simulink model "TP2"  (R2024b)
settings: Solver=VariableStepAuto  StartTime=0.0  StopTime=10  RelTol=1e-3
InitFcn:
  | J=0.28 %kg.m2.s-2
  | b=8.5e-3 %N.m.s
  | K=0.5093 %N.m.A-1
  | R=0.13 %Omh
  | L=1.6e-3 %H
  | Cr=0 %N.m
  | U=12 %V
  | v=2 %m.s-1
  | Kpos=1
StartFcn:
  | J=0.28 %kg.m2.s-2
  | b=8.5e-3 %N.m.s
  | K=0.5093 %N.m.A-1
  | R=0.13 %Omh
  | L=1.6e-3 %H
  | Cr=0 %N.m
  | U=12 %V
  | v=2 %m.s-1
  | Kpos=1
settings Model: Creator=E306-PC5  LastModifiedBy=E306-PC5

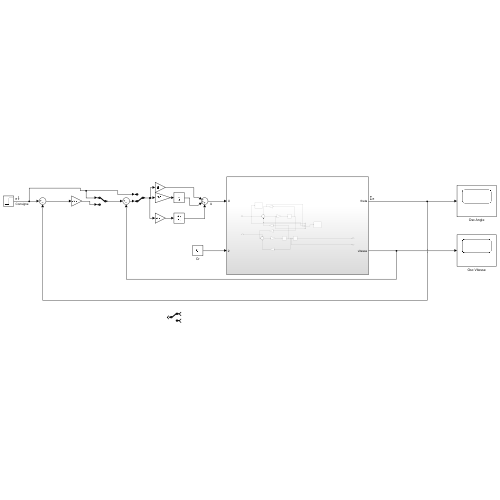
[thumbnail: Simulink's stored preview of the top-level diagram]
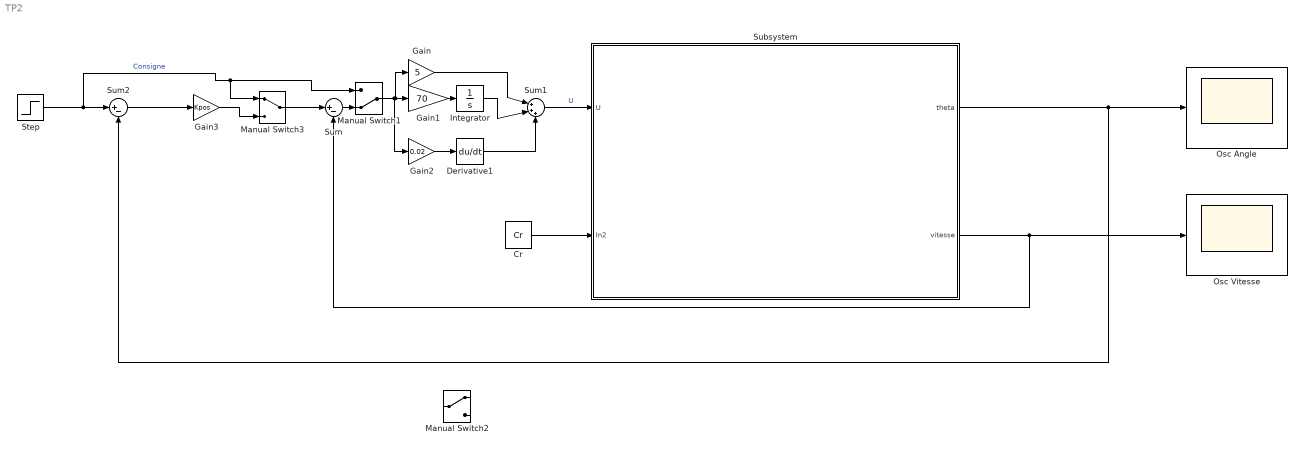
== system TP2 ==
  Cr : Constant  Value=Cr
  Derivative1 : Derivative
  Gain : Gain  Gain=5
  Gain1 : Gain  Gain=70
  Gain2 : Gain  Gain=0.02
  Gain3 : Gain  Gain=Kpos
  Integrator : Integrator
  Manual Switch1 : ManualSwitch  CurrentSetting=0
  Manual Switch2 : ManualSwitch
  Manual Switch3 : ManualSwitch
  Osc Angle : Scope
  Osc Vitesse : Scope
  Step : Step  Time=0.1  After=v  SampleTime=0
  Subsystem : Subsystem
  Sum : Sum  Inputs=|+-
  Sum1 : Sum  Inputs=|+++
  Sum2 : Sum  Inputs=|+-
  wires:
  Cr/1 -> Subsystem/2(In2)
  Subsystem/2(vitesse) -> Sum/2, Osc Vitesse/1
  Gain/1 -> Sum1/1
  Gain1/1 -> Integrator/1
  Integrator/1 -> Sum1/2
  Gain2/1 -> Derivative1/1
  Derivative1/1 -> Sum1/3
  Manual Switch1/1 -> Gain2/1, Gain/1, Gain1/1
  Sum/1 -> Manual Switch1/2
  Subsystem/1(theta) -> Sum2/2, Osc Angle/1
  Sum1/1 -> Subsystem/1(U)  "U"
  Step/1 -> Manual Switch3/1, Manual Switch1/1, Sum2/1  "Consigne"
  Sum2/1 -> Gain3/1
  Gain3/1 -> Manual Switch3/2
  Manual Switch3/1 -> Sum/1

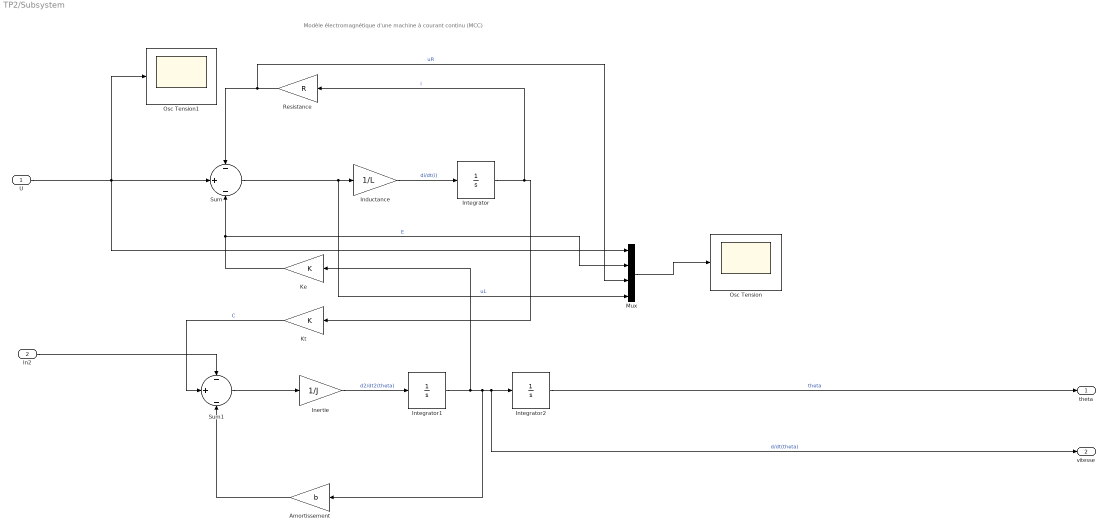
== system TP2/Subsystem ==
  note: Modèle électromagnétique d'une machine à courant continu (MCC)
  U : Inport
  In2 : Inport  Port=2
  Amortissement : Gain  Gain=b
  Inductance : Gain  Gain=1/L
  Inertie : Gain  Gain=1/J
  Integrator : Integrator
  Integrator1 : Integrator
  Integrator2 : Integrator
  Ke : Gain  Gain=K
  Kt : Gain  Gain=K
  Mux : Mux
  Osc Tension : Scope
  Osc Tension1 : Scope
  Resistance : Gain  Gain=R
  Sum : Sum  Inputs=-|+|-
  Sum1 : Sum  Inputs=-|+|-
  theta : Outport
  vitesse : Outport  Port=2
  wires:
  In2/1 -> Sum1/1
  Resistance/1 -> Mux/3, Sum/1  "uR"
  Ke/1 -> Sum/3, Mux/2  "E"
  Inductance/1 -> Integrator/1  "di/dt(i)"
  Sum/1 -> Mux/4, Inductance/1  "uL"
  Integrator/1 -> Resistance/1, Kt/1  "i"
  Integrator1/1 -> Ke/1, Amortissement/1, vitesse/1, Integrator2/1  "d/dt(theta)"
  Sum1/1 -> Inertie/1
  Inertie/1 -> Integrator1/1  "d2/dt2(theta)"
  U/1 -> Osc Tension1/1, Mux/1, Sum/2
  Amortissement/1 -> Sum1/3
  Kt/1 -> Sum1/2  "C"
  Integrator2/1 -> theta/1  "theta"
  Mux/1 -> Osc Tension/1
